simulink model "Am_Complete"  (Simulink 7.7)
settings: Solver=FixedStepDiscrete  StartTime=0.0  StopTime=0.524288  FixedStep=2e-6  RelTol=1e-3
undefined symbols (not defined in the file or in its folder): dfilt, fdesignblkfcn, gcbh, get, One, sided
libraries: dspsrcs4 x5, dsparch4 x4, dspsnks4 x3, commchan3 x1
settings Model: Creator=ArunKB  LastModifiedBy=ArunKB

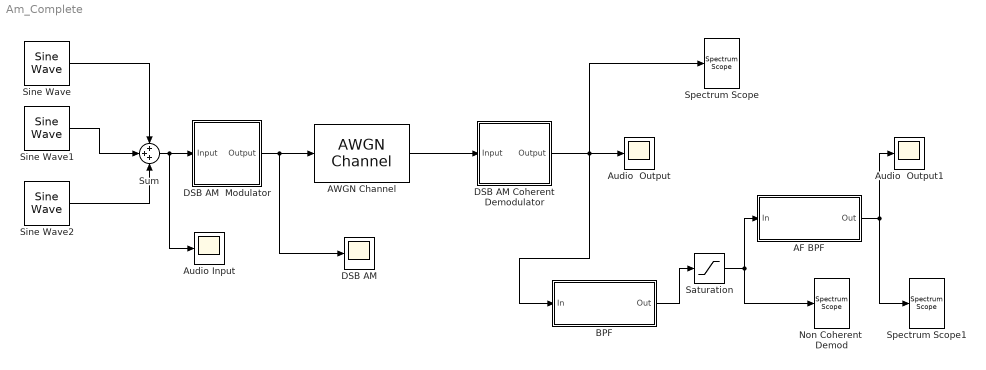
== system Am_Complete ==
  AF BPF : Subsystem  DialogController=fdesignblkfcn  DialogControllerArgs=DataTag1  InitFcn=fdesignblkfcn(gcbh, {'InitFcn'});
      settings: CopyFcn=fdesignblkfcn(gcbh, {'CopyFcn'});
      mask Type: Bandpass Filter
      mask Description: Design a bandpass filter
      mask Help: helpview(mapfilelocation('dsp'), 'dspbandpassfilter');
      mask Display: disp('Bandpass');
  AWGN Channel : commchan3/AWGN Channel  SystemSampleTime=-1  InputProcessing=Columns as channels (frame based)  seed=67  noiseMode=Variance from mask  EbNodB=10  EsNodB=10  SNRdB=10  bitsPerSym=1  Ps=1  Tsym=1  variance=1
  Audio  Output : Scope
      settings: TimeRange=0.01400000000000001  YMin=-3  YMax=3  SaveName=ScopeData2
  Audio  Output1 : Scope
      settings: TimeRange=0.01400000000000001  YMin=-3  YMax=3  SaveName=ScopeData3
  Audio Input : Scope
      settings: TimeRange=0.01400000000000001  YMin=-3  YMax=3
  BPF : Subsystem  DialogController=fdesignblkfcn  DialogControllerArgs=DataTag5  InitFcn=fdesignblkfcn(gcbh, {'InitFcn'});
      settings: CopyFcn=fdesignblkfcn(gcbh, {'CopyFcn'});
      mask Type: Bandpass Filter
      mask Description: Design a bandpass filter
      mask Help: helpview(mapfilelocation('dsp'), 'dspbandpassfilter');
      mask Display: disp('Bandpass');
  DSB AM : Scope
      settings: TimeRange=0.01400000000000001  YMin=-30  YMax=30
  DSB AM  Modulator : Subsystem
  DSB AM Coherent Demodulator : Subsystem
  Non Coherent  Demod : dspsnks4/Spectrum Scope  SystemSampleTime=-1  ScopeProperties=on  Domain=Frequency  HorizSpan=1  UseBuffer=on  BufferSize=262144  Overlap=0  TreatMby1Signals=One channel  inpFftLenInherit=on  FFTlength=262144  numAvg=1  DisplayProperties=off  AxisGrid=on  Memory=off  FrameNumber=on  AxisLegend=off  AxisZoom=off  OpenScopeAtSimStart=on  OpenScopeImmediately=off  FigPos=get(0,'defaultfigureposition')  AxisProperties=off  XUnits=Hertz  XRange=One-sided ([0...Fs/2])  XDisplay=0  InheritXIncr=on  XIncr=1.0  XLabel=Samples  XLimit=User-defined  YUnits=dBW/Hertz  XMax=50965.7118  XMin=-28.2118  YLabel=Magnitude-squared, dB  LineProperties=off  wintypeSpecScope=Boxcar  RsSpecScope=50  betaSpecScope=5  winsampSpecScope=Periodic  XAxisParamsVer=6.9  isFrameUpgraded=on
      settings: YMin=-417.5279  YMax=-285.2417
  Saturation : Saturate  UpperLimit=1000  LowerLimit=0
  Sine Wave : dspsrcs4/Sine Wave  Amplitude=1  Frequency=500  Phase=0  SampleMode=Discrete  OutComplex=Real  CompMethod=Trigonometric fcn  TableSize=Speed  SampleTime=2e-6  SamplesPerFrame=1  ResetState=Restart at time zero  dataType=double  wordLen=16  udDataType=sfix(16)  fracBitsMode=Best precision  numFracBits=15  OutDataTypeStr=double  LastOutDataTypeStr=double
  Sine Wave1 : dspsrcs4/Sine Wave  Amplitude=1  Frequency=1500  Phase=0  SampleMode=Discrete  OutComplex=Real  CompMethod=Trigonometric fcn  TableSize=Speed  SampleTime=2e-6  SamplesPerFrame=1  ResetState=Restart at time zero  dataType=double  wordLen=16  udDataType=sfix(16)  fracBitsMode=Best precision  numFracBits=15  OutDataTypeStr=double  LastOutDataTypeStr=double
  Sine Wave2 : dspsrcs4/Sine Wave  Amplitude=1  Frequency=2500  Phase=0  SampleMode=Discrete  OutComplex=Real  CompMethod=Trigonometric fcn  TableSize=Speed  SampleTime=2e-6  SamplesPerFrame=1  ResetState=Restart at time zero  dataType=double  wordLen=16  udDataType=sfix(16)  fracBitsMode=Best precision  numFracBits=15  OutDataTypeStr=double  LastOutDataTypeStr=double
  Spectrum Scope : dspsnks4/Spectrum Scope  SystemSampleTime=-1  ScopeProperties=on  Domain=Frequency  HorizSpan=1  UseBuffer=on  BufferSize=262144  Overlap=0  TreatMby1Signals=One channel  inpFftLenInherit=on  FFTlength=262144  numAvg=1  DisplayProperties=off  AxisGrid=on  Memory=off  FrameNumber=on  AxisLegend=off  AxisZoom=off  OpenScopeAtSimStart=on  OpenScopeImmediately=off  FigPos=get(0,'defaultfigureposition')  AxisProperties=off  XUnits=Hertz  XRange=One-sided ([0...Fs/2])  XDisplay=0  InheritXIncr=on  XIncr=1.0  XLabel=Samples  XLimit=User-defined  YUnits=dBW/Hertz  XMax=50965.7118  XMin=-28.2118  YLabel=Magnitude-squared, dB  LineProperties=off  wintypeSpecScope=Boxcar  RsSpecScope=50  betaSpecScope=5  winsampSpecScope=Periodic  XAxisParamsVer=6.9  isFrameUpgraded=on
      settings: YMin=-128.2795  YMax=2.7316
  Spectrum Scope1 : dspsnks4/Spectrum Scope  SystemSampleTime=-1  ScopeProperties=on  Domain=Frequency  HorizSpan=1  UseBuffer=on  BufferSize=262144  Overlap=0  TreatMby1Signals=One channel  inpFftLenInherit=on  FFTlength=262144  numAvg=1  DisplayProperties=off  AxisGrid=on  Memory=off  FrameNumber=on  AxisLegend=off  AxisZoom=off  OpenScopeAtSimStart=on  OpenScopeImmediately=off  FigPos=get(0,'defaultfigureposition')  AxisProperties=off  XUnits=Hertz  XRange=One-sided ([0...Fs/2])  XDisplay=0  InheritXIncr=on  XIncr=1.0  XLabel=Samples  XLimit=User-defined  YUnits=dBW/Hertz  XMax=50965.7118  XMin=-28.2118  YLabel=Magnitude-squared, dB  LineProperties=off  wintypeSpecScope=Boxcar  RsSpecScope=50  betaSpecScope=5  winsampSpecScope=Periodic  XAxisParamsVer=6.9  isFrameUpgraded=on
      settings: YMin=-433.5071  YMax=-300.3135
  Sum : Sum  Inputs=+++
  wires:
  DSB AM  Modulator/1(Output) -> AWGN Channel/1, DSB AM/1
  AWGN Channel/1 -> DSB AM Coherent Demodulator/1(Input)
  DSB AM Coherent Demodulator/1(Output) -> Audio  Output/1, Spectrum Scope/1, BPF/1(In)
  AF BPF/1(Out) -> Spectrum Scope1/1, Audio  Output1/1
  Saturation/1 -> AF BPF/1(In), Non Coherent  Demod/1
  BPF/1(Out) -> Saturation/1
  Sine Wave1/1 -> Sum/2
  Sum/1 -> DSB AM  Modulator/1(Input), Audio Input/1
  Sine Wave2/1 -> Sum/3
  Sine Wave/1 -> Sum/1

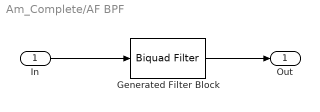
== system Am_Complete/AF BPF ==
  In : Inport
  Generated Filter Block : dsparch4/Biquad Filter  Tag=BlockMethodSubSystem  IIRFiltStruct=Direct form II  CoeffSource=Specify via dialog  BiQuadCoeffs=[0.0291297897468329 0 -0.0291297897468329 1 -1.99322618838867 0.993438686870846;0.00122953524862917 0 -0.00122953524862917 1 -1.99216650501323 0.993207275696802;0.00114178304940285 0 -0.00114178304940285 1 -1.99958375308644 0.999615921104786;0.0451568518312421 0 -0.0451568518312421 1 -1.99856595776928 0.998609444767157;0.119741544592112 0 -0.119741544592112 1 -1.99092763126749 0.991477782666749;0.00457449418724176 0 -0.00457449418724176 1 -1.9960478896537 0.997458461978987;2 0 -2 1 -1.99662062910845 0.996702756858355]  a0Flag=Warning  IC=0  ICnum=0  ICden=0  InputProcessing=Columns as channels (frame based)  denAccumFracLength=30  denProdOutputFracLength=30  secondMemoryFracLength=15  roundingMode=Floor  overflowMode=off  ScaleValues=[9.33403539464049e-005;1;1;1;1;1;1;43.4351912222513]  optimizeScaleValues=off  ScaleValueMode=Specify via input port (g)  scaleValueFracLength=14  FilterSource=Specify via dialog  dfiltObjectName=dfilt.df2tsos([1 0.3 0.4],[1 0.1 0.2])
  Out : Outport
  wires:
  Generated Filter Block/1 -> Out/1
  In/1 -> Generated Filter Block/1

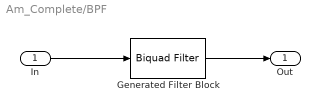
== system Am_Complete/BPF ==
  In : Inport
  Generated Filter Block : dsparch4/Biquad Filter  Tag=BlockMethodSubSystem  IIRFiltStruct=Direct form II  CoeffSource=Specify via dialog  BiQuadCoeffs=[0.003484185766584 0 -0.003484185766584 1 -1.95849823522399 0.997548270388572;0.0273305288694723 0 -0.0273305288694723 1 -1.95627601669044 0.996588886211245;0.103816079266736 0 -0.103816079266736 1 -1.94329652344671 0.993198528015041;0.0462937256046046 0 -0.0462937256046046 1 -1.91283894794366 0.992985528724662;0.08022159604534 0 -0.08022159604534 1 -1.9347268934232 0.992109484051246;0.120331130920276 0 -0.120331130920276 1 -1.92098093016611 0.991915252908046;0.0105709117033808 0 -0.0105709117033808 1 -1.90706639790271 0.994994704165103;0.00331947797200272 0 -0.00331947797200272 1 -1.95058002800878 0.994765464209076;0.14506267782667 0 -0.14506267782667 1 -1.9616879807767 0.999506809219698;0.13709489108513 0 -0.13709489108513 1 -1.90524561020689 0.99922811504808;0.007952368140749 0 -0.007952368140749 1 -1.90544913432174 0.996286425283002;0.0331815736403288 0 -0.0331815736403288 1 -1.95363505627936 0.995656117106807;0.0882233103509631 0 -0.0882233103509631 1 -1.93914127726063 0.99257827640947;0.0524403952368919 0 -0.0524403952368919 1 -1.91669801171737 0.992325905475786;0.0257429770543376 0 -0.0257429770543376 1 -1.93014609015539 0.99182452907933;0.0190413614742594 0 -0.0190413614742594 1 -1.925516948363 0.99175236683448;0.0705422112992775 0 -0.0705422112992775 1 -1.94712469131635 0.993937641232746;0.0175385107383816 0 -0.0175385107383816 1 -1.90957507086074 0.993882925096412;0.140349795408284 0 -0.140349795408284 1 -1.96030182684321 0.998523367097532;2 0 -2 1 -1.90482384457517 0.997714428986945]  a0Flag=Warning  IC=0  ICnum=0  ICden=0  InputProcessing=Columns as channels (frame based)  denAccumFracLength=30  denProdOutputFracLength=30  secondMemoryFracLength=15  roundingMode=Floor  overflowMode=off  ScaleValues=[0.000486714790797815;1;1;1;1;1;1;1;1;1;1;1;1;1;1;1;1;1;1;1;1.28326225879894]  optimizeScaleValues=off  ScaleValueMode=Specify via input port (g)  scaleValueFracLength=14  FilterSource=Specify via dialog  dfiltObjectName=dfilt.df2tsos([1 0.3 0.4],[1 0.1 0.2])
  Out : Outport
  wires:
  In/1 -> Generated Filter Block/1
  Generated Filter Block/1 -> Out/1

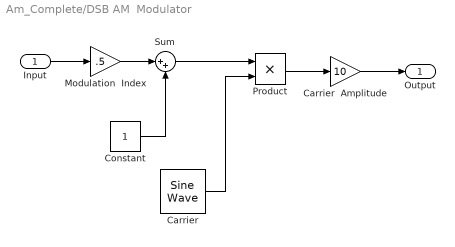
== system Am_Complete/DSB AM  Modulator ==
  Input : Inport
  Carrier : dspsrcs4/Sine Wave  Amplitude=1  Frequency=20000  Phase=0  SampleMode=Discrete  OutComplex=Real  CompMethod=Trigonometric fcn  TableSize=Speed  SampleTime=2e-6  SamplesPerFrame=1  ResetState=Restart at time zero  dataType=double  wordLen=16  udDataType=sfix(16)  fracBitsMode=Best precision  numFracBits=15  OutDataTypeStr=double  LastOutDataTypeStr=double
  Carrier  Amplitude : Gain  Gain=10
  Constant : Constant
  Modulation  Index : Gain  Gain=.5
  Product : Product  RndMeth=Zero
  Sum : Sum  Inputs=|++
  Output : Outport
  wires:
  Input/1 -> Modulation  Index/1
  Modulation  Index/1 -> Sum/1
  Constant/1 -> Sum/2
  Sum/1 -> Product/1
  Carrier/1 -> Product/2
  Product/1 -> Carrier  Amplitude/1
  Carrier  Amplitude/1 -> Output/1

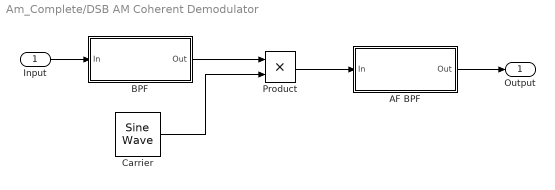
== system Am_Complete/DSB AM Coherent Demodulator ==
  Input : Inport
  AF BPF : Subsystem  DialogController=fdesignblkfcn  DialogControllerArgs=DataTag8  InitFcn=fdesignblkfcn(gcbh, {'InitFcn'});
      settings: CopyFcn=fdesignblkfcn(gcbh, {'CopyFcn'});
      mask Type: Bandpass Filter
      mask Description: Design a bandpass filter
      mask Help: helpview(mapfilelocation('dsp'), 'dspbandpassfilter');
      mask Display: disp('Bandpass');
  BPF : Subsystem  DialogController=fdesignblkfcn  DialogControllerArgs=DataTag11  InitFcn=fdesignblkfcn(gcbh, {'InitFcn'});
      settings: CopyFcn=fdesignblkfcn(gcbh, {'CopyFcn'});
      mask Type: Bandpass Filter
      mask Description: Design a bandpass filter
      mask Help: helpview(mapfilelocation('dsp'), 'dspbandpassfilter');
      mask Display: disp('Bandpass');
  Carrier : dspsrcs4/Sine Wave  Amplitude=1  Frequency=20000  Phase=0  SampleMode=Discrete  OutComplex=Real  CompMethod=Trigonometric fcn  TableSize=Speed  SampleTime=2e-6  SamplesPerFrame=1  ResetState=Restart at time zero  dataType=double  wordLen=16  udDataType=sfix(16)  fracBitsMode=Best precision  numFracBits=15  OutDataTypeStr=double  LastOutDataTypeStr=double
  Product : Product  RndMeth=Zero
  Output : Outport
  wires:
  Input/1 -> BPF/1(In)
  BPF/1(Out) -> Product/1
  Product/1 -> AF BPF/1(In)
  AF BPF/1(Out) -> Output/1
  Carrier/1 -> Product/2

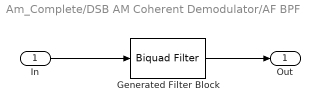
== system Am_Complete/DSB AM Coherent Demodulator/AF BPF ==
  In : Inport
  Generated Filter Block : dsparch4/Biquad Filter  Tag=BlockMethodSubSystem  IIRFiltStruct=Direct form II  CoeffSource=Specify via dialog  BiQuadCoeffs=[0.0310111828269258 0 -0.0310111828269258 1 -1.99533379437818 0.999274615607648;0.00884828415152441 0 -0.00884828415152441 1 -1.99908834329562 0.999143058884078;0.0278136228176343 0 -0.0278136228176343 1 -1.99250415930458 0.995375654923485;0.0179368576695061 0 -0.0179368576695061 1 -1.99442682038231 0.994889484476812;0.0220844793530578 0 -0.0220844793530578 1 -1.99212938247417 0.993850128523829;0.00189687665647024 0 -0.00189687665647024 1 -1.99247745904989 0.993671743816194;0.0299423704868057 0 -0.0299423704868057 1 -1.99411433927677 0.997856584106322;0.031007817472344 0 -0.031007817472344 1 -1.99706858719754 0.997232430693178;0.0309924091345846 0 -0.0309924091345846 1 -1.99990256883058 0.999934580066434;0.0196512044384585 0 -0.0196512044384585 1 -1.99976276398928 0.999796449252563;0.00613578099491103 0 -0.00613578099491103 1 -1.99865745246339 0.998730560855247;0.101054245281818 0 -0.101054245281818 1 -1.99801320123577 0.998118508444676;0.0144306903260581 0 -0.0144306903260581 1 -1.99215206563645 0.99445209089483;0.00797881338346703 0 -0.00797881338346703 1 -1.99324799682852 0.994015462871248;0.0290946667678021 0 -0.0290946667678021 1 -1.9931635008713 0.996534881749289;0.0303542053330218 0 -0.0303542053330218 1 -1.99581024442104 0.996082003543708;0.00303063276540821 0 -0.00303063276540821 1 -1.99959739791386 0.999634764334984;2 0 -2 1 -1.99938393808609 0.999427784845794]  a0Flag=Warning  IC=0  ICnum=0  ICden=0  InputProcessing=Columns as channels (frame based)  denAccumFracLength=30  denProdOutputFracLength=30  secondMemoryFracLength=15  roundingMode=Floor  overflowMode=off  ScaleValues=[4.71437257875915e-005;1;1;1;1;1;1;1;1;1;1;1;1;1;1;1;1;1;40.7367214311324]  optimizeScaleValues=off  ScaleValueMode=Specify via input port (g)  scaleValueFracLength=14  FilterSource=Specify via dialog  dfiltObjectName=dfilt.df2tsos([1 0.3 0.4],[1 0.1 0.2])
  Out : Outport
  wires:
  Generated Filter Block/1 -> Out/1
  In/1 -> Generated Filter Block/1

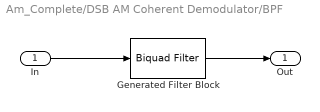
== system Am_Complete/DSB AM Coherent Demodulator/BPF ==
  In : Inport
  Generated Filter Block : dsparch4/Biquad Filter  Tag=BlockMethodSubSystem  IIRFiltStruct=Direct form II  CoeffSource=Specify via dialog  BiQuadCoeffs=[0.003484185766584 0 -0.003484185766584 1 -1.95849823522399 0.997548270388572;0.0273305288694723 0 -0.0273305288694723 1 -1.95627601669044 0.996588886211245;0.103816079266736 0 -0.103816079266736 1 -1.94329652344671 0.993198528015041;0.0462937256046046 0 -0.0462937256046046 1 -1.91283894794366 0.992985528724662;0.08022159604534 0 -0.08022159604534 1 -1.9347268934232 0.992109484051246;0.120331130920276 0 -0.120331130920276 1 -1.92098093016611 0.991915252908046;0.0105709117033808 0 -0.0105709117033808 1 -1.90706639790271 0.994994704165103;0.00331947797200272 0 -0.00331947797200272 1 -1.95058002800878 0.994765464209076;0.14506267782667 0 -0.14506267782667 1 -1.9616879807767 0.999506809219698;0.13709489108513 0 -0.13709489108513 1 -1.90524561020689 0.99922811504808;0.007952368140749 0 -0.007952368140749 1 -1.90544913432174 0.996286425283002;0.0331815736403288 0 -0.0331815736403288 1 -1.95363505627936 0.995656117106807;0.0882233103509631 0 -0.0882233103509631 1 -1.93914127726063 0.99257827640947;0.0524403952368919 0 -0.0524403952368919 1 -1.91669801171737 0.992325905475786;0.0257429770543376 0 -0.0257429770543376 1 -1.93014609015539 0.99182452907933;0.0190413614742594 0 -0.0190413614742594 1 -1.925516948363 0.99175236683448;0.0705422112992775 0 -0.0705422112992775 1 -1.94712469131635 0.993937641232746;0.0175385107383816 0 -0.0175385107383816 1 -1.90957507086074 0.993882925096412;0.140349795408284 0 -0.140349795408284 1 -1.96030182684321 0.998523367097532;2 0 -2 1 -1.90482384457517 0.997714428986945]  a0Flag=Warning  IC=0  ICnum=0  ICden=0  InputProcessing=Columns as channels (frame based)  denAccumFracLength=30  denProdOutputFracLength=30  secondMemoryFracLength=15  roundingMode=Floor  overflowMode=off  ScaleValues=[0.000486714790797815;1;1;1;1;1;1;1;1;1;1;1;1;1;1;1;1;1;1;1;1.28326225879894]  optimizeScaleValues=off  ScaleValueMode=Specify via input port (g)  scaleValueFracLength=14  FilterSource=Specify via dialog  dfiltObjectName=dfilt.df2tsos([1 0.3 0.4],[1 0.1 0.2])
  Out : Outport
  wires:
  In/1 -> Generated Filter Block/1
  Generated Filter Block/1 -> Out/1
